simulink model "week3_traffic_light"  (R2020a)
settings: Solver=VariableStepAuto  StartTime=0.0  StopTime=200  RelTol=1e-3
settings Model: Creator=Prateek  LastModifiedBy=Prateek

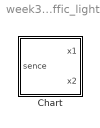
== system week3_traffic_light ==
  Chart : Stateflow chart  TreatAsAtomicUnit=on

== stateflow chart week3_traffic_light/Chart ==
  state stop
    x1=red;
    x2=green;
  state stopForTraffic
    x1=red;
    x2=green;
  state stopToGo
    x1=red;
    x2=yellow;
  state goToStop
    x1=yellow;
    x2=red;
  state go
    x1=green;
    x2=red;
  (default) -> stop
  stopForTraffic -> stopToGo : [sence]
  stop -> stopForTraffic : after(20,tick)
  stopToGo -> go : after(3,tick)
  goToStop -> stop : after(3,tick)
  go -> goToStop : after(10,tick)
  data: sence input; x1 output; x2 output; red local; yellow local; green local
